simulink model "problem1_simulink"  (R2017b)
settings: Solver=ode4  StartTime=0.0  StopTime=tfinal  FixedStep=h  RelTol=1e-3
libraries: cstblocks x6
settings Model: Creator=ameyadike  LastModifiedBy=Rahul Vivek Sawant
settings CodeAppCC: StateflowObjectComments=on

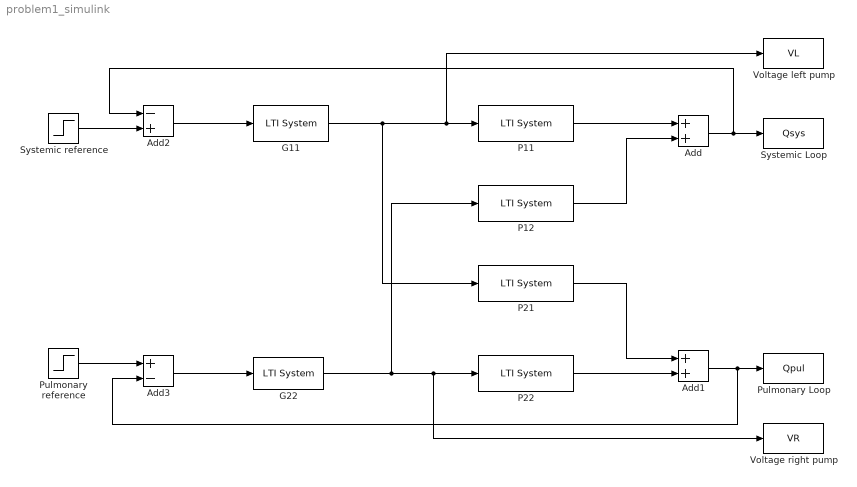
== system problem1_simulink ==
  Add : Sum
  Add1 : Sum
  Add2 : Sum  Inputs=-+
  Add3 : Sum  Inputs=+-
  G11 : cstblocks/LTI System  sys=G11  IC=[]
  G22 : cstblocks/LTI System  sys=G22  IC=[]
  P11 : cstblocks/LTI System  sys=P11  IC=[]
  P12 : cstblocks/LTI System  sys=P12  IC=[]
  P21 : cstblocks/LTI System  sys=P21  IC=[]
  P22 : cstblocks/LTI System  sys=P22  IC=[]
  Pulmonary Loop : ToWorkspace  VariableName=Qpul  SampleTime=-1
  Pulmonary reference : Step  Time=20  Before=4  After=6  SampleTime=0
  Systemic Loop : ToWorkspace  VariableName=Qsys  SampleTime=-1
  Systemic reference : Step  Time=10  Before=4  After=5  SampleTime=0
  Voltage left pump : ToWorkspace  VariableName=VL  SampleTime=-1
  Voltage right pump : ToWorkspace  VariableName=VR  SampleTime=-1
  wires:
  P11/1 -> Add/1
  P22/1 -> Add1/2
  P12/1 -> Add/2
  P21/1 -> Add1/1
  G11/1 -> P21/1, Voltage left pump/1, P11/1
  G22/1 -> P12/1, Voltage right pump/1, P22/1
  Systemic reference/1 -> Add2/2
  Pulmonary reference/1 -> Add3/1
  Add2/1 -> G11/1
  Add3/1 -> G22/1
  Add1/1 -> Pulmonary Loop/1, Add3/2
  Add/1 -> Systemic Loop/1, Add2/1
